simulink model "PthSet_OvrRunCoord"  (R2016b)
settings: configuration reference "CodeGenConfigSet" (kept outside this file)
values from neighbouring files (symbols this model uses):
  PthSet_trqOvrRunThres_C = Calibration.Parameter    [init_PthSet_OvrRunCoord.m]
  TRQ_ZERO = fi(0,Trq_Nm)    [init_PthSet_OvrRunCoord.m]
undefined symbols (not defined in the file or in its folder): EngState_conv
settings Model: Creator=Wollf  LastModifiedBy=Wollf
settings ConfigSetRef: SourceLocation=Base Workspace

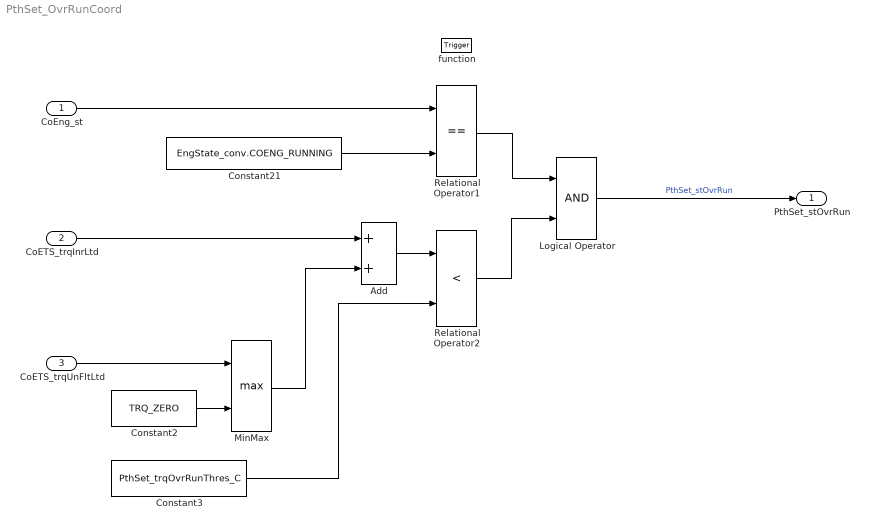
== system PthSet_OvrRunCoord ==
  CoEng_st : Inport  Description=Engine coordinator state  OutDataTypeStr=Enum: EngState_conv
  CoETS_trqInrLtd : Inport  Tag=Nm  Description=inner torque set value after limitation, before AS  Port=2  OutMin=-3000  OutMax=3000  OutDataTypeStr=Trq_Nm
  CoETS_trqUnFltLtd : Inport  Tag=Nm  Description=Limited idle speed governor torque  Port=3  OutMin=-3276  OutMax=3276  OutDataTypeStr=Trq_Nm
  function : TriggerPort  TriggerType=function-call  VariantControl=Variant
  Add : Sum  InputSameDT=on
  Constant2 : Constant  Value=TRQ_ZERO  OutDataTypeStr=Trq_Nm
  Constant21 : Constant  Value=EngState_conv.COENG_RUNNING  OutDataTypeStr=Inherit: Inherit via back propagation
  Constant3 : Constant  Value=PthSet_trqOvrRunThres_C
  Logical Operator : Logic  OutDataTypeStr=boolean
  MinMax : MinMax  Function=max  Inputs=2  InputSameDT=on
  Relational Operator1 : RelationalOperator  Operator===  OutDataTypeStr=boolean  RndMeth=Simplest  InputSameDT=on
  Relational Operator2 : RelationalOperator  Operator=<  OutDataTypeStr=boolean  RndMeth=Simplest  InputSameDT=on
  PthSet_stOvrRun : Outport  Description=State of overrun detection (0: No overrun; 1: overrun)  OutMin=0  OutMax=1  OutDataTypeStr=boolean
  wires:
  Constant2/1 -> MinMax/2
  MinMax/1 -> Add/2
  CoETS_trqInrLtd/1 -> Add/1
  Constant3/1 -> Relational Operator2/2
  CoEng_st/1 -> Relational Operator1/1
  Constant21/1 -> Relational Operator1/2
  CoETS_trqUnFltLtd/1 -> MinMax/1
  Add/1 -> Relational Operator2/1
  Relational Operator2/1 -> Logical Operator/2
  Logical Operator/1 -> PthSet_stOvrRun/1  "PthSet_stOvrRun"
  Relational Operator1/1 -> Logical Operator/1
